simulink model "calc"  (R2021a)
settings: Solver=FixedStepDiscrete  StartTime=0.0  StopTime=10.0  RelTol=1e-3  EnableMultiTasking=on
libraries: simulink x2
settings Model: Creator=Noha  LastModifiedBy=Noha
settings DataIOCC: ReturnWorkspaceOutputs=off
settings OptimizationCC: DefaultParameterBehavior=Inlined  InlineInvariantSignals=on  EnableMemcpy=off  LifeSpan=1  EfficientTunableParamExpr=on
settings DebuggingCC: UnderspecifiedInitializationDetection=Classic  MergeDetectMultiDrivingBlocksExec=none  SFMachineParentedDataDiag=warning  ArithmeticOperatorsInVariantConditions=warning
settings ModelReferenceCC: PropagateSignalLabelsOutOfModel=off
settings SFSimCC: MATLABDynamicMemAlloc=off  CustomCodeUndefinedFunction=UseInterfaceOnly
settings RTWCC: SystemTargetFile=ert.tlc  GenCodeOnly=on  TemplateMakefile=ert_default_tmf  GenerateReport=on  IncludeHyperlinkInReport=on  LaunchReport=on  GenerateTraceInfo=on  GenerateTraceReport=on  GenerateTraceReportSl=on  GenerateTraceReportSf=on  GenerateTraceReportEml=on
settings CodeAppCC: ForceParamTrailComments=on  IgnoreCustomStorageClasses=off  OperatorAnnotations=on  SimulinkDataObjDesc=on  SFDataObjDesc=on  MATLABFcnDesc=on  InsertBlockDesc=on  StateflowObjectComments=on  MATLABSourceComments=on
settings ERTTargetCC: MultiwordLength=2048  GenerateSampleERTMain=on  InlinedParameterPlacement=NonHierarchical  ERTCustomFileTemplate=example_file_process.tlc

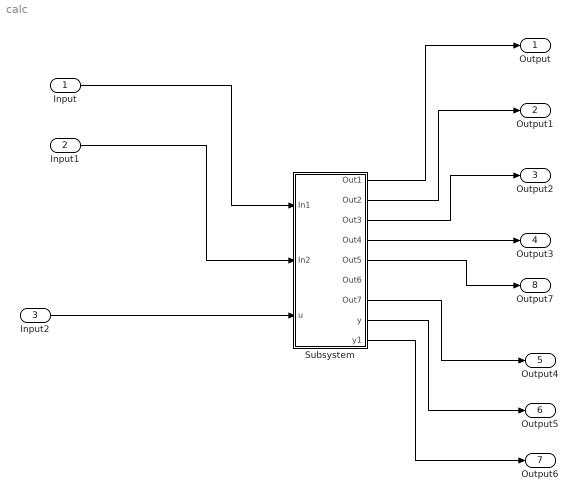
== system calc ==
  Input : Inport
  Input1 : Inport  Port=2
  Input2 : Inport  Port=3
  Subsystem : Subsystem
  Output : Outport
  Output1 : Outport  Port=2
  Output2 : Outport  Port=3
  Output3 : Outport  Port=4
  Output4 : Outport  Port=5
  Output5 : Outport  Port=6
  Output6 : Outport  Port=7
  Output7 : Outport  Port=8
  wires:
  Input/1 -> Subsystem/1(In1)
  Input1/1 -> Subsystem/2(In2)
  Input2/1 -> Subsystem/3(u)
  Subsystem/1(Out1) -> Output/1
  Subsystem/2(Out2) -> Output1/1
  Subsystem/3(Out3) -> Output2/1
  Subsystem/4(Out4) -> Output3/1
  Subsystem/5(Out5) -> Output7/1
  Subsystem/7(Out7) -> Output4/1
  Subsystem/8(y) -> Output5/1
  Subsystem/9(y1) -> Output6/1

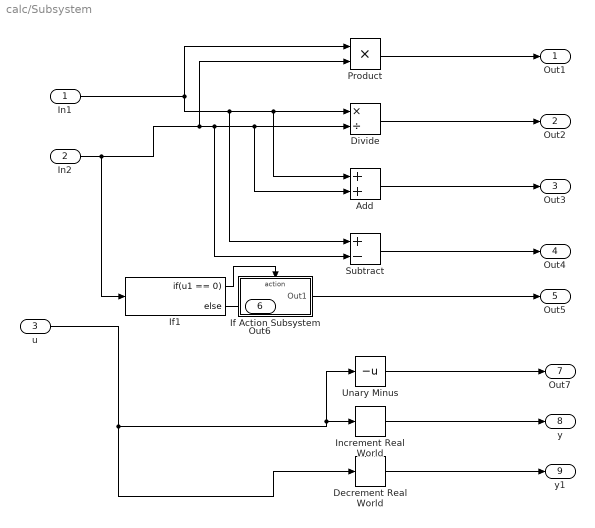
== system calc/Subsystem ==
  In1 : Inport
  In2 : Inport  Port=2
  u : Inport  Port=3
  Add : Sum
  Decrement Real World : simulink/Additional Math & Discrete/Additional Math: Increment - Decrement/Decrement Real World
      settings: SourceProductBaseCode=SL
  Divide : Product  Inputs=*/
  If Action Subsystem : Subsystem  TreatAsAtomicUnit=on
  If1 : If  IfExpression=u1 == 0
  Increment Real World : simulink/Additional Math & Discrete/Additional Math: Increment - Decrement/Increment Real World
      settings: SourceProductBaseCode=SL
  Product : Product
  Subtract : Sum  Inputs=+-
  Unary Minus : UnaryMinus
  Out1 : Outport
  Out2 : Outport  Port=2
  Out3 : Outport  Port=3
  Out4 : Outport  Port=4
  Out5 : Outport  Port=5
  Out6 : Outport  Port=6
  Out7 : Outport  Port=7
  y : Outport  Port=8
  y1 : Outport  Port=9
  wires:
  In1/1 -> Subtract/1, Add/1, Divide/1, Product/1
  Add/1 -> Out3/1
  In2/1 -> If1/1, Product/2, Subtract/2, Add/2, Divide/2
  Divide/1 -> Out2/1
  Unary Minus/1 -> Out7/1
  u/1 -> Decrement Real World/1, Unary Minus/1, Increment Real World/1
  If1/1 -> If Action Subsystem/Action
  If Action Subsystem/1(Out1) -> Out5/1
  Product/1 -> Out1/1
  Subtract/1 -> Out4/1
  Increment Real World/1 -> y/1
  Decrement Real World/1 -> y1/1
  If1/2 -> Out6/1

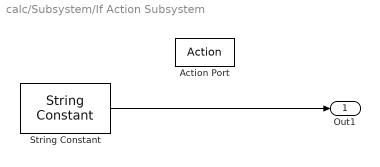
== system calc/Subsystem/If Action Subsystem ==
  Action Port : ActionPort  ActionPortLabel=if(u1 == 0)
  String Constant : StringConstant  String="\"not vaild div by zero\""
  Out1 : Outport
  wires:
  String Constant/1 -> Out1/1
